simulink model "mpclinearization"  (Simulink 7.2)
settings: Solver=ode45  StartTime=0.0  StopTime=10.0  RelTol=1e-3
libraries: mpclib x1
Description:
  | MPC Control Design Using a Linearized Plant Model
  | 
  | This demo opens the Model Predictive Control Design Tool to tune an MPC controller for a nonlinear plant in Simulink(R).  If Simulink(R) Control Design(TM) is installed, the MPC internal model will be obtained from linearization of the plant model.
settings Model: Creator=jowen  LastModifiedBy=rchen
settings SolverCC: ZeroCrossAlgorithm=Non-adaptive
settings DataIOCC: SignalLoggingName=logsOut
settings OptimizationCC: InlineInvariantSignals=on  InitFltsAndDblsToZero=on  EfficientMapNaN2IntZero=off
settings DebuggingCC: SaveWithParameterizedLinksMsg=none  CheckExecutionContextPreStartOutputMsg=on  CheckExecutionContextRuntimeOutputMsg=on  SignalResolutionControl=TryResolveAllWithWarning  SolverPrmCheckMsg=none  MultiTaskDSMMsg=warning  MultiTaskCondExecSysMsg=none  StrictBusMsg=None
settings RTWCC: IncludeERTFirstTime=on
settings CodeAppCC: MangleLength=5
settings GRTTargetCC: TargetFcnLib=ansi_tfl_tmw.mat

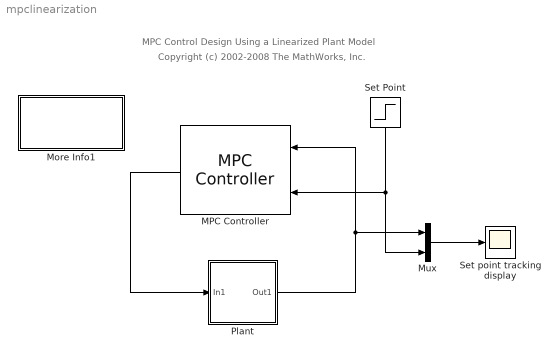
== system mpclinearization ==
  note: MPC Control Design Using a Linearized Plant Model
  note: Copyright (c) 2002-2008 The MathWorks, Inc.
  MPC Controller : mpclib/MPC Controller  Orientation=left  SystemSampleTime=-1  n_mv=1  x0=[]  ref_from_ws=off  ref_signal_name=[]  ref_preview=on  md_from_ws=off  md_signal_name=[]  md_preview=on  from_project=off  md_inport=off  mv_inport=off  lims_inport=off  switch_inport=off  enable_value=0  project_file=MPCtask.mat  is_multiple=0
  More Info1 : Subsystem
      settings: OpenFcn=mpcdesign_callback('mpclinearization')
      mask Display: disp('Double click\nhere to\nStart')
  Mux : Mux  Inputs=2
  Plant : Subsystem
  Set Point : Step  Orientation=down  SampleTime=0
  Set point tracking display : Scope
  wires:
  Plant/1(Out1) -> Mux/1, MPC Controller/1
  Set Point/1 -> Mux/2, MPC Controller/2
  Mux/1 -> Set point tracking display/1
  MPC Controller/1 -> Plant/1(In1)

== system mpclinearization/More Info1 ==

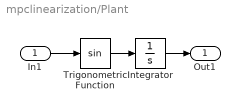
== system mpclinearization/Plant ==
  In1 : Inport  OutDataType=sfix(16)  OutScaling=2^0
  Integrator : Integrator
  Trigonometric Function : Trigonometry
  Out1 : Outport  OutDataType=sfix(16)  OutScaling=2^0
  wires:
  Trigonometric Function/1 -> Integrator/1
  Integrator/1 -> Out1/1
  In1/1 -> Trigonometric Function/1
